simulink model "mpptproject_solarcellsweep"  (R2025a)
settings: Solver=VariableStepAuto  StartTime=0.0  StopTime=1000  RelTol=1e-3
libraries: fl_lib x7, nesl_utility x6, ee_lib x1
settings Model: Creator=jacks  LastModifiedBy=jacks

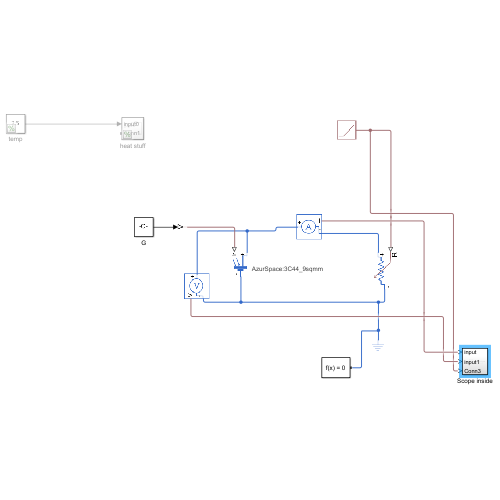
[thumbnail: Simulink's stored preview of the top-level diagram]
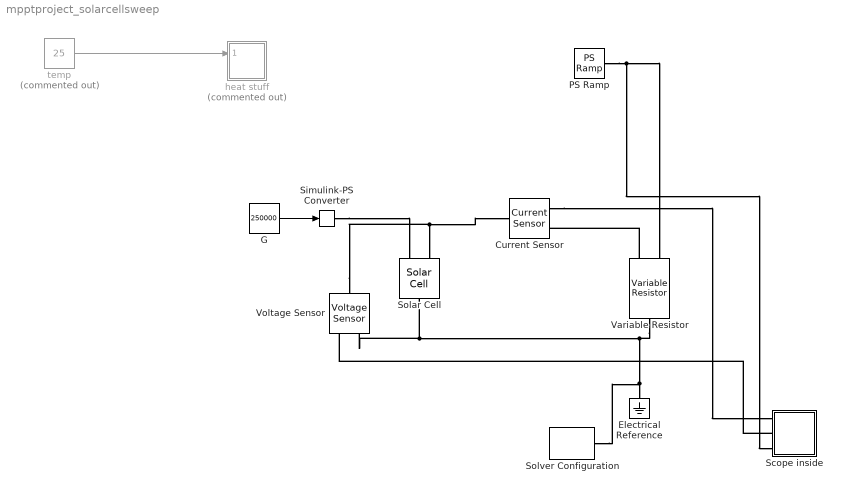
== system mpptproject_solarcellsweep ==
  Current Sensor : fl_lib/Electrical/Electrical Sensors/Current Sensor
  Electrical Reference : fl_lib/Electrical/Electrical Elements/Electrical Reference
  G : Constant  Value=250000
  PS Ramp : fl_lib/Physical Signals/Sources/PS Ramp  slope=0.2 1/s  start_time=0 s  initial_output=0.0000001  ZeroCross=true
  Scope inside : Subsystem
  Simulink-PS Converter : nesl_utility/Simulink-PS Converter  PhysicalDomain=network_engine_domain  SubClassName=ps_input  LeftPortType=input  RightPortType=output  PseudoPeriodic=off  Frequencies=[]  NoiseDistribution=none  NoiseParameters=[]  Unit=1  AffineConversion=off  FilteringAndDerivatives=provide  SimscapeFilterOrder=1  InputFilterTimeConstant=0.001  UdotUserProvided=0
  Solar Cell : ee_lib/Sources/Solar Cell  PartSpecification="{\"CollectionId\":\"SimscapeElectrical\",\"CollectionVersion\":\"1.0.0\",\"DatasetId\":\"AzurSpace|3C44_9sqmm|simscape.electrical.solarCell\",\"DisplayName\":\"AzurSpace:3C44_9sqmm\"}"  prm=3  Isc=0.37 % Datasheet derived A  Voc=3.05 % Datasheet derived V  Is=1.91003784590348e-35 % Datasheet derived A  Is2=8.42205890783812e-38 % Datasheet derived A  Iph=0.370001258541474 % Datasheet derived A  Ir0=250000 % Datasheet derived W/m^2  ec=1.50364371134548 % Datasheet derived  N2=1.73316940278898 % Datasheet derived  Rs=0.306625056084457 % Datasheet derived Ohm  Rp=90147.3159723304 % Datasheet derived Ohm  N_series=1 % Datasheet derived  N_parallel=1 % Datasheet derived  TIPH1=0.000800010328673928 % Datasheet derived 1/K  EG=1.441 % Datasheet derived eV  TXIS1=104.115941100637 % Datasheet derived  TXIS2=5.57230100941371 % Datasheet derived  TRS1=0.775797800706674 % Datasheet derived  TRP1=0 % Parameter not set  Tmeas=25 % Datasheet derived degC  TFIXED=25 % Datasheet derived degC  thermal_mass=100 % Parameter not set J/K  initial_temperature=25 degC
      settings: AttributesFormatString=AzurSpace:3C44_9sqmm
  Solver Configuration : nesl_utility/Solver Configuration  PhysicalDomain=network_engine_domain  SubClassName=solver  LeftPortType=input  RightPortType=generic  Tones=[]  Harmonics=[]  SimulateNoise=off  Profile=off  UseLocalSampling=off  EnableSwitchedLinearOptims=on  FrequencyDomain=off  UseCCode=off  RelTol=0.001  AbsTol=0.001  MinStep=1e-09  ToWorkspace=off  RevertToSquareIcSolve=off  NumHomotopyIterations=100  PhasorMode=off  PhasorModeNumHarmonics=1  ConsistencySolver=NEWTON_XTOL_AFTER_FTOL  IndexReductionMethod=DerivativeReplacement  DoDC=off  ResidualTolerance=1e-09  ConsistencyTolSource=GLOBAL  ConsistencyAbsTol=0.001  ConsistencyRelTol=0.001  ConsistencyTolFactor=0.001  UseLocalSolver=off  LocalSolverChoice=NE_BACKWARD_EULER_ADVANCER  ResolveIndetEquations=on  FunctionEvalNumThread=1  LocalSolverSampleTime=0.001  DoFixedCost=off  MaxNonlinIter=3  MaxModeIter=2  ComputeImpulses=off  ImpulseIterations=2  LinearAlgebra=auto  LinearAlgebraNumThread=0  EquationFormulation=NE_TIME_EF  DelaysMemoryBudget=1024  AutomaticFiltering=on  FilteringTimeConstant=0.001  PartitionStorageMethod=AS_NEEDED  PartitionMemoryBudget=1024  PartitionMethod=ROBUST  MultibodyUseLocalSolver=off  MultibodyLocalSolverChoice=ODE1  MultibodyLocalSolverSampleTime=0.001
  Variable Resistor : fl_lib/Electrical/Electrical Elements/Variable Resistor  Rmin=0 Ohm  thermalEnable=false  thermal_mass=1 J/K  i_specify=off  i_priority=None  i=0 A  i_nominal_specify=off  i_nominal_value=1  i_nominal_unit=A  v_specify=off  v_priority=None  v=0 V  v_nominal_specify=off  v_nominal_value=1  v_nominal_unit=V  T_specify=off  T_priority=None  T=300 K  T_nominal_specify=off  T_nominal_value=1  T_nominal_unit=K
  Voltage Sensor : fl_lib/Electrical/Electrical Sensors/Voltage Sensor
  heat stuff : Subsystem  Commented=on
  temp : Constant  Commented=on  Value=25
  wires:
  G/1 -> Simulink-PS Converter/1
  temp/1 -> heat stuff/1(input0)
  connections:
  Simulink-PS Converter/RConn1 -- Solar Cell/LConn1
  Voltage Sensor/RConn2 -- Variable Resistor/RConn1 -- Solver Configuration/RConn1 -- Electrical Reference/LConn1 -- Solar Cell/RConn1
  Voltage Sensor/LConn1 -- Current Sensor/LConn1 -- Solar Cell/LConn2
  PS Ramp/RConn1 -- Scope inside/LConn3 -- Variable Resistor/LConn1
  Current Sensor/RConn1 -- Scope inside/LConn1
  Scope inside/LConn2 -- Voltage Sensor/RConn1
  Variable Resistor/LConn2 -- Current Sensor/RConn2

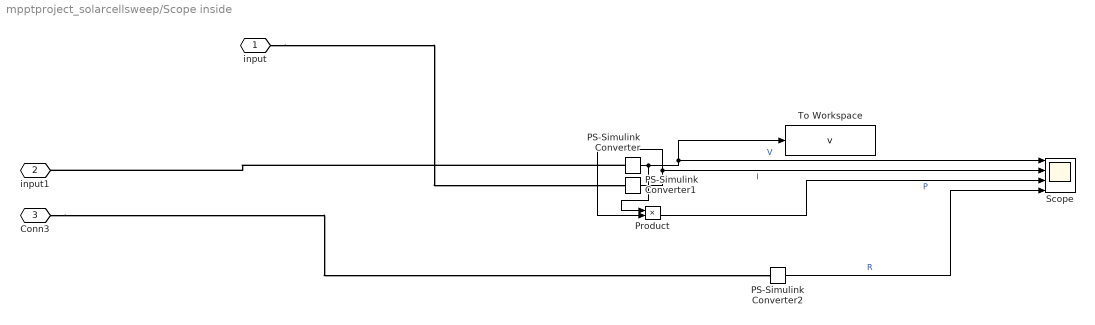
== system mpptproject_solarcellsweep/Scope inside ==
  PS-Simulink Converter : nesl_utility/PS-Simulink Converter  PhysicalDomain=network_engine_domain  SubClassName=ps_output  LeftPortType=input  RightPortType=output  PseudoPeriodic=off  Frequencies=[]  VectorFormat=inherit  Unit=V  AffineConversion=off
  PS-Simulink Converter1 : nesl_utility/PS-Simulink Converter  PhysicalDomain=network_engine_domain  SubClassName=ps_output  LeftPortType=input  RightPortType=output  PseudoPeriodic=off  Frequencies=[]  VectorFormat=inherit  Unit=A  AffineConversion=off
  PS-Simulink Converter2 : nesl_utility/PS-Simulink Converter  PhysicalDomain=network_engine_domain  SubClassName=ps_output  LeftPortType=input  RightPortType=output  PseudoPeriodic=off  Frequencies=[]  VectorFormat=inherit  Unit=A  AffineConversion=off
  Product : Product
  Scope : Scope  NumInputPorts=4
      settings: ActiveDisplayYMinimum=-0.39727575295760742  ActiveDisplayYMaximum=6.7428710496257347
  To Workspace : ToWorkspace  VariableName=v  SaveFormat=Timeseries  SampleTime=-1
  input : PMIOPort  Side=Left
  input1 : PMIOPort  Port=2  Side=Left
  Conn3 : PMIOPort  Port=3  Side=Left
  wires:
  PS-Simulink Converter/1 -> Product/1, To Workspace/1, Scope/1  "V"
  PS-Simulink Converter1/1 -> Product/2, Scope/2  "I"
  Product/1 -> Scope/3  "P"
  PS-Simulink Converter2/1 -> Scope/4  "R"
  connections:
  PS-Simulink Converter/LConn1 -- input1/RConn1
  input/RConn1 -- PS-Simulink Converter1/LConn1
  Conn3/RConn1 -- PS-Simulink Converter2/LConn1

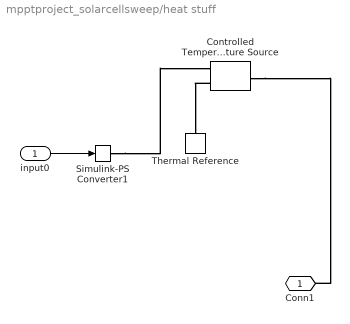
== system mpptproject_solarcellsweep/heat stuff ==
  input0 : Inport
  Controlled Temperature Source : fl_lib/Thermal/Thermal Sources/Controlled Temperature Source
  Simulink-PS Converter1 : nesl_utility/Simulink-PS Converter  PhysicalDomain=network_engine_domain  SubClassName=ps_input  LeftPortType=input  RightPortType=output  PseudoPeriodic=off  Frequencies=[]  NoiseDistribution=none  NoiseParameters=[]  Unit=1  AffineConversion=off  FilteringAndDerivatives=provide  SimscapeFilterOrder=1  InputFilterTimeConstant=0.001  UdotUserProvided=0
  Thermal Reference : fl_lib/Thermal/Thermal Elements/Thermal Reference
  Conn1 : PMIOPort  Side=Left
  wires:
  input0/1 -> Simulink-PS Converter1/1
  connections:
  Controlled Temperature Source/RConn2 -- Thermal Reference/LConn1
  Simulink-PS Converter1/RConn1 -- Controlled Temperature Source/RConn1
  Controlled Temperature Source/LConn1 -- Conn1/RConn1
